simulink model "symulink3"  (Simulink 7.2)
settings: Solver=ode45  StartTime=0.0  StopTime=20  RelTol=1e-3
values from neighbouring files (symbols this model uses):
  k11 = 0.35    [GlobalParam.m]
  k12 = -0.5    [GlobalParam.m]
  k21 = -0.36    [GlobalParam.m]
  k22 = .36    (= 0.36)    [GlobalParam.m]
  k3 = -2    [GlobalParam.m]
settings Model: Creator=ALan  LastModifiedBy=ALan

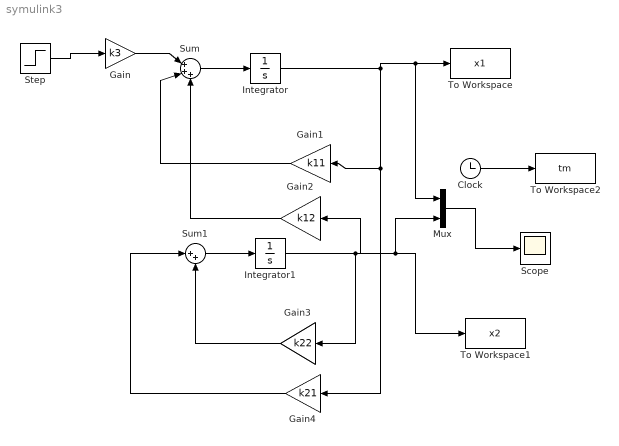
== system symulink3 ==
  Clock : Clock
      settings: Decimation=10
  Gain : Gain  Gain=k3  ParameterDataType=sfix(16)  ParameterScaling=2^0  OutDataType=sfix(16)  OutScaling=2^0
  Gain1 : Gain  Orientation=left  Gain=k11  ParameterDataType=sfix(16)  ParameterScaling=2^0  OutDataType=sfix(16)  OutScaling=2^0
  Gain2 : Gain  Orientation=left  Gain=k12  ParameterDataType=sfix(16)  ParameterScaling=2^0  OutDataType=sfix(16)  OutScaling=2^0
  Gain3 : Gain  Orientation=left  Gain=k22  ParameterDataType=sfix(16)  ParameterScaling=2^0  OutDataType=sfix(16)  OutScaling=2^0
  Gain4 : Gain  Orientation=left  Gain=k21  ParameterDataType=sfix(16)  ParameterScaling=2^0  OutDataType=sfix(16)  OutScaling=2^0
  Integrator : Integrator  InitialCondition=-3
  Integrator1 : Integrator  InitialCondition=-2
  Mux : Mux  Inputs=2
  Scope : Scope
  Step : Step  SampleTime=0
  Sum : Sum  Inputs=|+++  OutDataType=sfix(16)  OutScaling=2^0
  Sum1 : Sum  Inputs=|++  OutDataType=sfix(16)  OutScaling=2^0
  To Workspace : ToWorkspace  VariableName=x1  SampleTime=-1  SaveFormat=Array
  To Workspace1 : ToWorkspace  VariableName=x2  SampleTime=-1  SaveFormat=Array
  To Workspace2 : ToWorkspace  VariableName=tm  SampleTime=-1  SaveFormat=Array
  wires:
  Gain/1 -> Sum/1
  Sum/1 -> Integrator/1
  Integrator/1 -> Gain1/1, Gain4/1, To Workspace/1, Mux/1
  Gain1/1 -> Sum/2
  Sum1/1 -> Integrator1/1
  Integrator1/1 -> Gain2/1, Gain3/1, To Workspace1/1, Mux/2
  Gain2/1 -> Sum/3
  Gain3/1 -> Sum1/2
  Gain4/1 -> Sum1/1
  Step/1 -> Gain/1
  Clock/1 -> To Workspace2/1
  Mux/1 -> Scope/1
